simulink model "WDGBrakingLogic_Harness"  (R2024a)
settings: configuration reference "csMultiInstance" (kept outside this file)
undefined symbols (not defined in the file or in its folder): BrStatus
settings Model: DataDictionary=DD_WDGBrakingLogic.sldd  Creator=The MathWorks, Inc.  LastModifiedBy=The MathWorks, Inc.
settings ConfigSetRef: SourceName=csMultiInstance

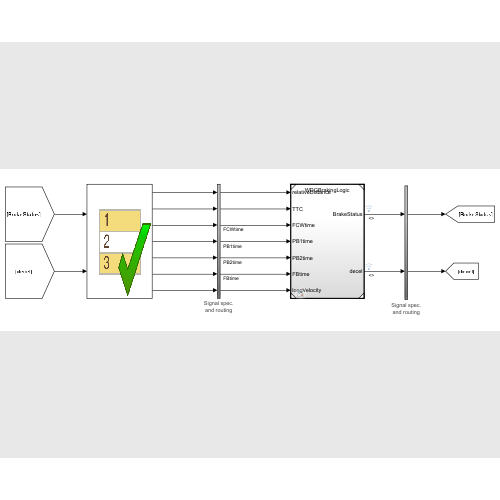
[thumbnail: Simulink's stored preview of the top-level diagram]
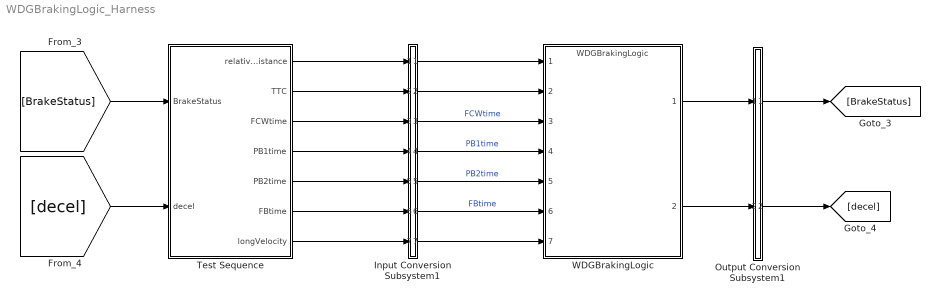
== system WDGBrakingLogic_Harness ==
  Input Conversion Subsystem1 : Subsystem  Tag=__SLT_ICS__  Description=|
      | Signal spec.
      | and routing
      settings: AttributesFormatString=%<Description>
  Output Conversion Subsystem1 : Subsystem  Tag=__SLT_OCS__  Description=|
      | Signal spec.
      | and routing
      settings: AttributesFormatString=%<Description>
  Test Sequence : Test Sequence  TreatAsAtomicUnit=on
  WDGBrakingLogic : ModelReference  ModelNameDialog=WDGBrakingLogic  SimulationMode=Normal  ModelReferenceVersion=7.0
  wires:
  [BrakeStatus] -> Test Sequence/1(BrakeStatus)
  [decel] -> Test Sequence/2(decel)
  WDGBrakingLogic/1 -> Output Conversion Subsystem1/1(Inport_1)
  Input Conversion Subsystem1/6(Outport_6) -> WDGBrakingLogic/6  "FBtime"
  Output Conversion Subsystem1/2(Outport_2) -> [decel]
  Input Conversion Subsystem1/7(Outport_7) -> WDGBrakingLogic/7
  WDGBrakingLogic/2 -> Output Conversion Subsystem1/2(Inport_2)
  Input Conversion Subsystem1/3(Outport_3) -> WDGBrakingLogic/3  "FCWtime"
  Test Sequence/2(TTC) -> Input Conversion Subsystem1/2(Inport_2)
  Input Conversion Subsystem1/4(Outport_4) -> WDGBrakingLogic/4  "PB1time"
  Input Conversion Subsystem1/1(Outport_1) -> WDGBrakingLogic/1
  Test Sequence/7(longVelocity) -> Input Conversion Subsystem1/7(Inport_7)
  Input Conversion Subsystem1/5(Outport_5) -> WDGBrakingLogic/5  "PB2time"
  Test Sequence/3(FCWtime) -> Input Conversion Subsystem1/3(Inport_3)
  Input Conversion Subsystem1/2(Outport_2) -> WDGBrakingLogic/2
  Output Conversion Subsystem1/1(Outport_1) -> [BrakeStatus]
  Test Sequence/5(PB2time) -> Input Conversion Subsystem1/5(Inport_5)
  Test Sequence/1(relativeDistance) -> Input Conversion Subsystem1/1(Inport_1)
  Test Sequence/6(FBtime) -> Input Conversion Subsystem1/6(Inport_6)
  Test Sequence/4(PB1time) -> Input Conversion Subsystem1/4(Inport_4)

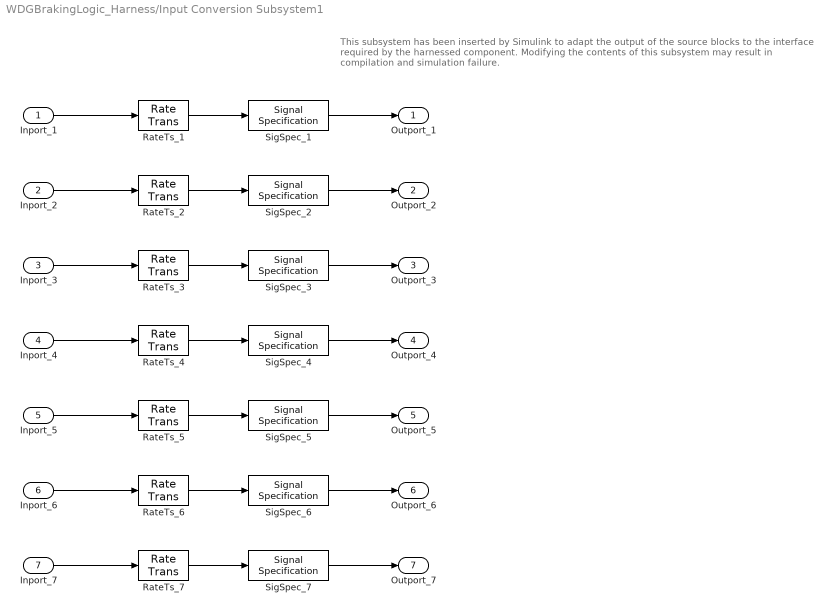
== system WDGBrakingLogic_Harness/Input Conversion Subsystem1 ==
  note: This subsystem has been inserted by Simulink to adapt the output of the source blocks to the interface required by the harnessed component.
      |  Modifying the contents of this subsystem may result in compilation and simulation failure.
  Inport_1 : Inport
  Inport_2 : Inport  Port=2
  Inport_3 : Inport  Port=3
  Inport_4 : Inport  Port=4
  Inport_5 : Inport  Port=5
  Inport_6 : Inport  Port=6
  Inport_7 : Inport  Port=7
  RateTs_{1..7} (7 alike) : RateTransition  OutPortSampleTime=0.1
  SigSpec_1 : SignalSpecification  OutDataTypeStr=double  Unit=m  Dimensions=[1]  SampleTime=0.1
  SigSpec_{2..6} (5 alike) : SignalSpecification  OutDataTypeStr=double  Unit=s  Dimensions=[1]  SampleTime=0.1
  SigSpec_7 : SignalSpecification  OutDataTypeStr=double  Unit=m/s  Dimensions=[1]  SampleTime=0.1
  Outport_1 : Outport
  Outport_2 : Outport  Port=2
  Outport_3 : Outport  Port=3
  Outport_4 : Outport  Port=4
  Outport_5 : Outport  Port=5
  Outport_6 : Outport  Port=6
  Outport_7 : Outport  Port=7
  wires:
  SigSpec_1/1 -> Outport_1/1
  RateTs_1/1 -> SigSpec_1/1
  Inport_1/1 -> RateTs_1/1
  SigSpec_2/1 -> Outport_2/1
  RateTs_2/1 -> SigSpec_2/1
  Inport_2/1 -> RateTs_2/1
  SigSpec_3/1 -> Outport_3/1
  RateTs_3/1 -> SigSpec_3/1
  Inport_3/1 -> RateTs_3/1
  SigSpec_4/1 -> Outport_4/1
  RateTs_4/1 -> SigSpec_4/1
  Inport_4/1 -> RateTs_4/1
  SigSpec_5/1 -> Outport_5/1
  RateTs_5/1 -> SigSpec_5/1
  Inport_5/1 -> RateTs_5/1
  SigSpec_6/1 -> Outport_6/1
  RateTs_6/1 -> SigSpec_6/1
  Inport_6/1 -> RateTs_6/1
  SigSpec_7/1 -> Outport_7/1
  RateTs_7/1 -> SigSpec_7/1
  Inport_7/1 -> RateTs_7/1

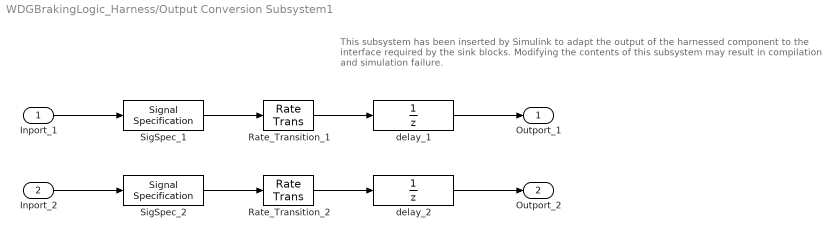
== system WDGBrakingLogic_Harness/Output Conversion Subsystem1 ==
  note: This subsystem has been inserted by Simulink to adapt the output of the harnessed component to the interface required by the sink blocks.
      |  Modifying the contents of this subsystem may result in compilation and simulation failure.
  Inport_1 : Inport
  Inport_2 : Inport  Port=2
  Rate_Transition_1 : RateTransition  InitialCondition=BrStatus.NoBrake  OutPortSampleTimeOpt=Inherit
  Rate_Transition_2 : RateTransition  OutPortSampleTimeOpt=Inherit
  SigSpec_1 : SignalSpecification  OutDataTypeStr=Enum: BrStatus  Dimensions=[1]  SampleTime=0.1
  SigSpec_2 : SignalSpecification  OutDataTypeStr=double  Unit=m/s^2  Dimensions=[1]  SampleTime=0.1
  delay_1 : UnitDelay  InitialCondition=BrStatus.NoBrake  SampleTime=-1
  delay_2 : UnitDelay  SampleTime=-1
  Outport_1 : Outport
  Outport_2 : Outport  Port=2
  wires:
  Inport_1/1 -> SigSpec_1/1
  SigSpec_1/1 -> Rate_Transition_1/1
  Rate_Transition_1/1 -> delay_1/1
  delay_1/1 -> Outport_1/1
  Inport_2/1 -> SigSpec_2/1
  SigSpec_2/1 -> Rate_Transition_2/1
  Rate_Transition_2/1 -> delay_2/1
  delay_2/1 -> Outport_2/1

== stateflow chart WDGBrakingLogic_Harness/Test Sequence ==
  state Run
    %% Initialize data outputs.
    relativeDistance = 90;
    TTC = -9;
    FCWtime = 7.95;
    PB1time = 7.11;
    PB2time = 5.09;
    FBtime = 2.76;
    longVelocity = 27;
  state step_1
    relativeDistance = 80;
    TTC = -8;
    FCWtime = 7.95;
    PB1time = 7.11;
    PB2time = 5.09;
    FBtime = 2.76;
    longVelocity = 27;
  state step_2
    relativeDistance = 70;
    TTC = -7;
    FCWtime = 7.95;
    PB1time = 7.11;
    PB2time = 5.09;
    FBtime = 2.76;
    longVelocity = 27;
  state step_3
    relativeDistance = 60;
    TTC = -6;
    FCWtime = 7.95;
    PB1time = 7.11;
    PB2time = 5.09;
    FBtime = 2.76;
    longVelocity = 27;
  state step_4
    relativeDistance = 50;
    TTC = -5;
    FCWtime = 7.95;
    PB1time = 7.11;
    PB2time = 5.09;
    FBtime = 2.76;
    longVelocity = 27;
  state step_5
    relativeDistance = 40;
    TTC = -4;
    FCWtime = 7.95;
    PB1time = 7.11;
    PB2time = 5.09;
    FBtime = 2.76;
    longVelocity = 27;
  state step_6
    relativeDistance = 30;
    TTC = -3;
    FCWtime = 7.95;
    PB1time = 7.11;
    PB2time = 5.09;
    FBtime = 2.76;
    longVelocity = 27;
  state step_7
    relativeDistance = 20;
    TTC = -2;
    FCWtime = 7.95;
    PB1time = 7.11;
    PB2time = 5.09;
    FBtime = 2.76;
    longVelocity = 27;
  state step_8
    relativeDistance = 10;
    TTC = -1;
    FCWtime = 7.95;
    PB1time = 7.11;
    PB2time = 5.09;
    FBtime = 2.76;
    longVelocity = 27;
  state step_9
    relativeDistance = 8;
    TTC = -8;
    FCWtime = 7.95;
    PB1time = 7.11;
    PB2time = 5.09;
    FBtime = 2.76;
    longVelocity = 27;
  (default) -> Run
  Run -> step_1 : [
      | after(1,'sec')
      | ]
  step_1 -> step_2 : [
      | after(1,'sec')
      | ]
  step_2 -> step_3 : [
      | after(1,'sec')
      | ]
  step_3 -> step_4 : [
      | after(1,'sec')
      | ]
  step_4 -> step_5 : [
      | after(1,'sec')
      | ]
  step_5 -> step_6 : [
      | after(1,'sec')
      | ]
  step_6 -> step_7 : [
      | after(1,'sec')
      | ]
  step_7 -> step_8 : [
      | after(1,'sec')
      | ]
  step_8 -> step_9 : [
      | after(1,'sec')
      | ]
  data: BrakeStatus input Enum: BrStatus size=[1]; decel input double size=[1]; relativeDistance output double size=[1]; TTC output double size=[1]; FCWtime output double size=[1]; PB1time output double size=[1]; PB2time output double size=[1]; FBtime output double size=[1]; longVelocity output double size=[1]
